simulink model "Sistema_Seguimiento_Tipo1_Con_Planta_Tipo_1"  (R2016a)
settings: Solver=VariableStepAuto  StartTime=0.0  StopTime=4  RelTol=1e-3
values from neighbouring files (symbols this model uses):
  A = [ - Ra/La 0 -Kb/(r*La); 0 0 1 ; Kt/(r*Meq) -K/Meq -Beq/Meq]    [Final_2021.m]
  B = [ 1/La ; 0 ; 0]    [Final_2021.m]
  C = [ 0 1 0 ]    [Final_2021.m]
  D = [ 0 ]    [Final_2021.m]
libraries: simulink x1
settings Model: Creator=Abel  LastModifiedBy=Abel

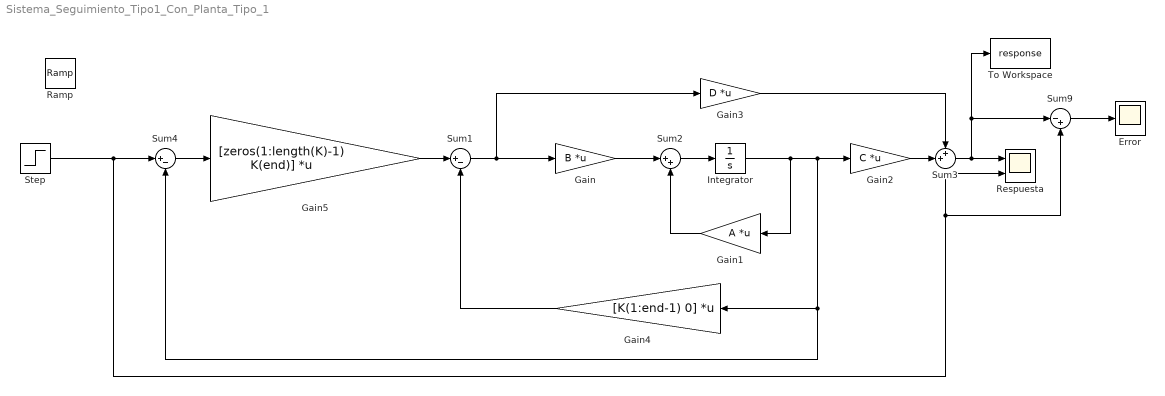
== system Sistema_Seguimiento_Tipo1_Con_Planta_Tipo_1 ==
  Error : Scope
  Gain : Gain  Gain=B  Multiplication=Matrix(K*u) (u vector)
  Gain1 : Gain  Gain=A  Multiplication=Matrix(K*u) (u vector)
  Gain2 : Gain  Gain=C  Multiplication=Matrix(K*u) (u vector)
  Gain3 : Gain  Gain=D  Multiplication=Matrix(K*u) (u vector)
  Gain4 : Gain  Gain=[K(1:end-1) 0]  Multiplication=Matrix(K*u) (u vector)
  Gain5 : Gain  Gain=[zeros(1:length(K)-1) K(end)]  Multiplication=Matrix(K*u) (u vector)
  Integrator : Integrator
  Ramp : simulink/Sources/Ramp  slope=1  start=0  X0=0
  Respuesta : Scope  NumInputPorts=2
  Step : Step  SampleTime=0
  Sum1 : Sum  Inputs=|+-
  Sum2 : Sum  Inputs=|++
  Sum3 : Sum  Inputs=++|
  Sum4 : Sum  Inputs=|+-
  Sum9 : Sum  Inputs=|-+
  To Workspace : ToWorkspace  VariableName=response  SaveFormat=Timeseries  SampleTime=-1
      settings: Save2DSignal=2-D array (concatenate along first dimension)
  wires:
  Sum1/1 -> Gain3/1, Gain/1
  Gain/1 -> Sum2/1
  Sum2/1 -> Integrator/1
  Gain1/1 -> Sum2/2
  Integrator/1 -> Sum4/2, Gain4/1, Gain2/1, Gain1/1
  Gain2/1 -> Sum3/2
  Gain3/1 -> Sum3/1
  Gain4/1 -> Sum1/2
  Gain5/1 -> Sum1/1
  Sum4/1 -> Gain5/1
  Sum3/1 -> Sum9/1, To Workspace/1, Respuesta/1
  Step/1 -> Sum9/2, Respuesta/2, Sum4/1
  Sum9/1 -> Error/1
